simulink library "APST_Lib"  (R2016a)
settings: Solver=ode45  StartTime=0.0  StopTime=10.0  RelTol=1e-3
undefined symbols (not defined in the file or in its folder): ACM, COMP_MAP, rev_comms_sink
libraries: APST_Lib x97
(part 5 of 6)

== system APST_Lib/Electrical Components/Load ==
  In1 : Inport
  In2 : Inport  Port=2
  Bus Selector : BusSelector  OutputSignals=V,I
  Constant : Constant  Value=0
  Constant1 : Constant  Value=0
  Data_Sink1 : APST_Lib/Support Components/Data_Sink
  Divide : Product  Inputs=/
  Gain : Gain  Gain=1000
  P : Constant  Value=P_max
  Product : Product
  Product1 : Product
  Sink1 : APST_Lib/Support Components/Sink
  Switch : Switch  Criteria=u2 > Threshold
  Switch1 : Switch  Criteria=u2 > Threshold
  Terminator3 : Terminator
  b1 : BusCreator  Inputs=1
  wires:
  Bus Selector/1 -> Switch1/2, Divide/1, Switch/2  "<V>"
  Bus Selector/2 -> Terminator3/1  "<I>"
  Product1/1 -> Gain/1  "I"
  In1/1 -> Bus Selector/1
  P/1 -> Product/1
  In2/1 -> Product/2
  Switch/1 -> Product1/1
  Divide/1 -> Switch/1
  Constant/1 -> Switch/3
  b1/1 -> Data_Sink1/1
  Switch1/1 -> b1/1, Product1/2  "Power"
  Constant1/1 -> Switch1/3
  Product/1 -> Switch1/1  "Power"
  Gain/1 -> Sink1/1

== system APST_Lib/Electrical Components/QLoad ==
  In1 : Inport
  In2 : Inport  Port=2
  Bus Selector : BusSelector  OutputSignals=V,I
  Constant : Constant  Value=0
  Constant1 : Constant  Value=0
  Data_Sink1 : APST_Lib/Support Components/Data_Sink
  Divide : Product  Inputs=/
  Divide1 : Product  Inputs=*/
  Fcn : Fcn  Expr=1-u
  Gain : Gain  Gain=1000
  P : Constant  Value=P_max
  Product : Product
  Product1 : Product
  Product2 : Product
  Sink1 : APST_Lib/Support Components/Sink
  Source1 : APST_Lib/Support Components/Source
  Switch : Switch  Criteria=u2 > Threshold
  Switch1 : Switch  Criteria=u2 > Threshold
  Terminator3 : Terminator
  b1 : BusCreator  Inputs=3
  b2 : BusCreator  Inputs=2
  eta : Fcn  Expr=a*u^2+b*u+c
  Out1 : Outport
  wires:
  Bus Selector/1 -> Divide/1, Switch/2, Switch1/2  "<V>"
  Bus Selector/2 -> Terminator3/1  "<I>"
  Product1/1 -> Gain/1  "I"
  In1/1 -> Bus Selector/1
  P/1 -> Product/1
  In2/1 -> Product/2
  Switch/1 -> Product1/1
  Divide/1 -> Switch/1
  Constant/1 -> Switch/3
  b1/1 -> Data_Sink1/1
  Switch1/1 -> b1/2, Divide1/1  "Power"
  b2/1 -> Out1/1
  [T] -> b2/1  "T"
  [Q] -> b2/2  "Q_kW"
  Source1/1 -> [T]
  [T] -> eta/1
  eta/1 -> b1/1, Fcn/1, Divide1/2  "eta"
  Divide1/1 -> Product1/2, Product2/1  "P_in"
  Product2/1 -> [Q]
  Fcn/1 -> Product2/2
  Constant1/1 -> Switch1/3
  Product/1 -> Switch1/1  "Power"
  [Q] -> b1/3  "Q_kW"
  Gain/1 -> Sink1/1

== system APST_Lib/Electrical Components/Switch ==
  In : Inport
  u : Inport  Port=2
  Bus Creator1 : BusCreator  Inputs=2
  Bus Selector : BusSelector  OutputSignals=V,I
  Product : Product
  Product1 : Product
  Sink1 : APST_Lib/Support Components/Sink
  Source1 : APST_Lib/Support Components/Source
  Terminator3 : Terminator
  Out : Outport
  wires:
  Product/1 -> Bus Creator1/1  "V"
  Bus Creator1/1 -> Out/1
  In/1 -> Bus Selector/1
  Product1/1 -> Sink1/1, Bus Creator1/2  "I"
  Bus Selector/2 -> Terminator3/1  "<I>"
  Bus Selector/1 -> Product/1  "<V>"
  u/1 -> Product1/1, Product/2
  Source1/1 -> Product1/2  "I"

== system APST_Lib/Source & Sinks/Flow Flow Source (Pressure) ==
  In2 : Inport
  In3 : Inport  Port=2
  Constant4 : Constant  Value=-1
  Source1 : Subsystem  mask(Source){}
      mask help: Used for receiving data from the downstream component.
      mask init:
      | n_src = gcb;
      | n_src = str2num(n_src(end));
      | try
      |     rev_comms_source(n_src);
      | catch
      | 
      | end
      mask Display: text(0.25,0.5,'Source')
  Terminator : Terminator
  b1 : BusCreator  Inputs=3
  Out1 : Outport
  wires:
  b1/1 -> Out1/1
  Constant4/1 -> b1/1  "mdot_kgps"
  In2/1 -> b1/2  "T_C"
  In3/1 -> b1/3  "P_kPa"
  Source1/1(Out1) -> Terminator/1

== system APST_Lib/Source & Sinks/Flow Sink (Generic) ==
  In4 : Inport
  In3 : Inport  Port=2
  Sink1 : APST_Lib/Support Components/Sink
  Terminator : Terminator
  wires:
  In3/1 -> Sink1/1
  In4/1 -> Terminator/1

== system APST_Lib/Source & Sinks/Flow Sink (Mass Flow Rate) ==
  In4 : Inport
  In3 : Inport  Port=2
  Sink1 : APST_Lib/Support Components/Sink
  Terminator : Terminator
  wires:
  In3/1 -> Sink1/1  "mdot_kgps"
  In4/1 -> Terminator/1

== system APST_Lib/Source & Sinks/Flow Sink (Pressure) ==
  In4 : Inport
  In3 : Inport  Port=2
  Sink1 : APST_Lib/Support Components/Sink
  Terminator : Terminator
  wires:
  In3/1 -> Sink1/1  "P_kPa"
  In4/1 -> Terminator/1

== system APST_Lib/Source & Sinks/Flow Source (Mass Flow Rate) ==
  In1 : Inport
  In2 : Inport  Port=2
  Constant4 : Constant  Value=-1
  Source1 : Subsystem  mask(Source){}
      mask help: Used for receiving data from the downstream component.
      mask init:
      | n_src = gcb;
      | n_src = str2num(n_src(end));
      | try
      |     rev_comms_source(n_src);
      | catch
      | 
      | end
      mask Display: text(0.25,0.5,'Source')
  Terminator : Terminator
  b1 : BusCreator  Inputs=3
  Out1 : Outport
  wires:
  b1/1 -> Out1/1
  In1/1 -> b1/2  "T_C"
  In2/1 -> b1/1  "mdot_kgps"
  Constant4/1 -> b1/3  "P_kPa"
  Source1/1(Out1) -> Terminator/1

== system APST_Lib/Support Components/Data Manager ==
  Data : Outport

== system APST_Lib/Support Components/Data_Sink ==
  " " : Inport
  tag scope: gdata_SupportComponentsData_Sink=global
  wires:
  " "/1 -> [gdata_SupportComponentsData_Sink]

== system APST_Lib/Support Components/Sink ==
  In1 : Inport
  tag scope: gdata_APST_LibSupportComponentsSink=global
  wires:
  In1/1 -> [gdata_APST_LibSupportComponentsSink]

== system APST_Lib/Support Components/Source ==
  Out1 : Outport
  wires:
  [gdata_Thermal_System_BUSM2FSink2] -> Out1/1

== system APST_Lib/Support Components/Unit Conversion  ==
  Signal_in : Inport
  conv_fcn : Fcn  Expr=(u(1)+459.67)/1.8-273.15
  Converted Signal Out : Outport
  wires:
  conv_fcn/1 -> Converted Signal Out/1
  Signal_in/1 -> conv_fcn/1

== system APST_Lib/Thermal Components/ACM Shaft  ==
  Power In/Out [vector] : Inport
  Bus Creator2 : BusCreator  Inputs=1
  Comp Inertia : Constant  Value=J_comp
  Data_Sink : APST_Lib/Support Components/Data_Sink
  Divide : Product  Inputs=*//
  Integrator : Integrator  InitialCondition=N_init * 2 * pi / 60 + eps  LimitOutput=on  LowerSaturationLimit=1e-3
  Mux : Mux
  Pwr Turb Inertia : Constant  Value=J_pcomp
  Shaft Inertia : Constant  Value=J_shaft
  Sum of Elements : Sum  Inputs=+
  Sum of Elements1 : Sum  Inputs=+
  Turb Inertia : Constant  Value=J_turb
  rad 2 rev : Gain  Gain=60/(2*pi)
  rad 2 rev1 : Gain  Gain=60/2/pi
  RPM : Outport
  wires:
  rad 2 rev/1 -> RPM/1
  Integrator/1 -> rad 2 rev/1, Divide/3, rad 2 rev1/1  "omega (rad/s)"
  Power In/Out [vector]/1 -> Sum of Elements/1
  Sum of Elements/1 -> Divide/1
  Divide/1 -> Integrator/1
  Sum of Elements1/1 -> Divide/2
  Shaft Inertia/1 -> Mux/1
  Comp Inertia/1 -> Mux/2
  Turb Inertia/1 -> Mux/3
  Pwr Turb Inertia/1 -> Mux/4
  Mux/1 -> Sum of Elements1/1
  rad 2 rev1/1 -> Bus Creator2/1  "RPM"
  Bus Creator2/1 -> Data_Sink/1

== system APST_Lib/Thermal Components/Air Volume ==
  In1 : Inport
  In2 : Inport  Port=2
  In3 : Inport  Port=3
  Air_Volume : MATLAB Function  TreatAsAtomicUnit=on
  Bus Creator2 : BusCreator  Inputs=3
  Bus Selector : BusSelector  OutputSignals=Q_kW
  Constant : Constant  Value=P_init
  Constant1 : Constant  Value=T_init
  Data_Sink1 : APST_Lib/Support Components/Data_Sink
  Demux : Demux  Outputs=3
  Integrate : Integrator  InitialCondition=[T_init P_init M_init]  LimitOutput=on
  Sink1 : APST_Lib/Support Components/Sink
  Sink2 : APST_Lib/Support Components/Sink  Commented=on
  Source1 : APST_Lib/Support Components/Source
  Terminator : Terminator
  b1 : BusCreator  Inputs=3
  gb1 : BusSelector  OutputSignals=mdot_kgps,T_C,P_kPa
  kW to W : Gain  Gain=1e3
  n-D Lookup Table1 : Lookup_n-D  BreakpointsForDimension1=Fluid.P  BreakpointsForDimension2=Fluid.T  BreakpointsForDimension3=[5, 7]  Table=Fluid.C_pt  ExtrapMethod=Clip  UseLastTableValue=on  RndMeth=Simplest  InputSameDT=on
  n-D Lookup Table2 : Lookup_n-D  BreakpointsForDimension1=Fluid.P  BreakpointsForDimension2=Fluid.T  BreakpointsForDimension3=[5, 7]  Table=Fluid.Rho_pt  ExtrapMethod=Clip  UseLastTableValue=on  RndMeth=Simplest  InputSameDT=on
  pout1 : From  Commented=on  GotoTag=T_tank
  Out1 : Outport
  wires:
  b1/1 -> Out1/1
  [Mdot_out] -> b1/1  "mdot_kgps"
  gb1/2 -> [T_in]  "<T_C>"
  [T_tank] -> b1/2  "T_C"
  gb1/1 -> [Mdot_in]  "<mdot_kgps>"
  In1/1 -> gb1/1
  [P_tank] -> b1/3  "P_kPa"
  gb1/3 -> Terminator/1  "<P_kPa>"
  [P_tank] -> Sink1/1
  Source1/1 -> [Mdot_out]
  In2/1 -> [T_amb]
  [Mdot_in] -> Air_Volume/2(Mdot_in)
  [Mdot_out] -> Air_Volume/3(Mdot_out)
  Air_Volume/1(x_dot) -> Integrate/1
  Integrate/1 -> Air_Volume/1(x), Demux/1
  Demux/1 -> [T_tank]
  Demux/2 -> [P_tank]
  Constant1/1 -> n-D Lookup Table2/2, n-D Lookup Table1/2
  Constant/1 -> n-D Lookup Table2/1, n-D Lookup Table1/1
  n-D Lookup Table1/1 -> Air_Volume/6(Cp)
  n-D Lookup Table2/1 -> Air_Volume/7(Rho)
  [T_in] -> Air_Volume/4(T_in)
  [T_amb] -> Air_Volume/5(T_amb)
  Bus Creator2/1 -> Data_Sink1/1
  [T_tank] -> Bus Creator2/1  "T"
  [P_tank] -> Bus Creator2/2  "P"
  [M_tank] -> Bus Creator2/3  "M"
  In3/1 -> Bus Selector/1
  kW to W/1 -> Air_Volume/8(Q)
  Demux/3 -> [M_tank]
  Bus Selector/1 -> kW to W/1  "<Q_kW>"
  pout1/1 -> Sink2/1

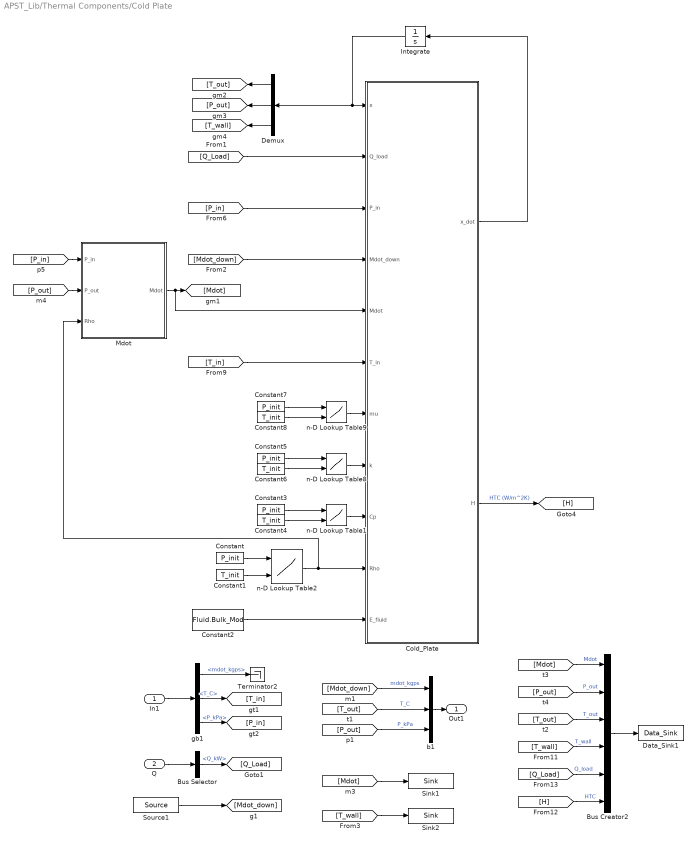
== system APST_Lib/Thermal Components/Cold Plate ==
  In1 : Inport
  Q : Inport  Port=2
  Bus Creator2 : BusCreator  Inputs=6
  Bus Selector : BusSelector  OutputSignals=Q_kW
  Cold_Plate : MATLAB Function  TreatAsAtomicUnit=on
  Constant{,3,5,7} (4 alike) : Constant  Value=P_init
  Constant{1,4,6,8} (4 alike) : Constant  Value=T_init
  Constant2 : Constant  Value=Fluid.Bulk_Mod
  Data_Sink1 : APST_Lib/Support Components/Data_Sink
  Demux : Demux  Outputs=3
  Integrate : Integrator  InitialCondition=[T_init P_init Tw_init]
  Mdot : MATLAB Function  TreatAsAtomicUnit=on
  Sink1 : APST_Lib/Support Components/Sink
  Sink2 : APST_Lib/Support Components/Sink
  Source1 : APST_Lib/Support Components/Source
  Terminator2 : Terminator
  b1 : BusCreator  Inputs=3
  gb1 : BusSelector  OutputSignals=mdot_kgps,T_C,P_kPa
  n-D Lookup Table1 : Lookup_n-D  BreakpointsForDimension1=Fluid.P  BreakpointsForDimension2=Fluid.T  BreakpointsForDimension3=[5, 7]  Table=Fluid.C_pt  ExtrapMethod=Clip  UseLastTableValue=on  RndMeth=Simplest  InputSameDT=on
  n-D Lookup Table2 : Lookup_n-D  BreakpointsForDimension1=Fluid.P  BreakpointsForDimension2=Fluid.T  BreakpointsForDimension3=[5, 7]  Table=Fluid.Rho_pt  ExtrapMethod=Clip  UseLastTableValue=on  RndMeth=Simplest  InputSameDT=on
  n-D Lookup Table8 : Lookup_n-D  BreakpointsForDimension1=Fluid.P  BreakpointsForDimension2=Fluid.T  BreakpointsForDimension3=[5, 7]  Table=Fluid.K_pt  ExtrapMethod=Clip  UseLastTableValue=on  RndMeth=Simplest  InputSameDT=on
  n-D Lookup Table9 : Lookup_n-D  BreakpointsForDimension1=Fluid.P  BreakpointsForDimension2=Fluid.T  BreakpointsForDimension3=[5, 7]  Table=Fluid.Mu_pt  ExtrapMethod=Clip  UseLastTableValue=on  RndMeth=Simplest  InputSameDT=on
  Out1 : Outport
  wires:
  Q/1 -> Bus Selector/1
  b1/1 -> Out1/1
  [Mdot_down] -> b1/1  "mdot_kgps"
  gb1/2 -> [T_in]  "<T_C>"
  [T_out] -> b1/2  "T_C"
  gb1/1 -> Terminator2/1  "<mdot_kgps>"
  In1/1 -> gb1/1
  [P_out] -> b1/3  "P_kPa"
  gb1/3 -> [P_in]  "<P_kPa>"
  [Mdot] -> Sink1/1
  [Q_Load] -> Cold_Plate/2(Q_load)
  Source1/1 -> [Mdot_down]
  [T_in] -> Cold_Plate/6(T_in)
  Cold_Plate/1(x_dot) -> Integrate/1
  Bus Creator2/1 -> Data_Sink1/1
  [T_wall] -> Bus Creator2/4  "T_wall"
  [T_out] -> Bus Creator2/3  "T_out"
  [P_out] -> Bus Creator2/2  "P_out"
  [Q_Load] -> Bus Creator2/5  "Q_load"
  [Mdot] -> Bus Creator2/1  "Mdot"
  Cold_Plate/2(H) -> [H]  "HTC (W/m^2K)"
  [H] -> Bus Creator2/6  "HTC"
  n-D Lookup Table8/1 -> Cold_Plate/8(k)
  n-D Lookup Table9/1 -> Cold_Plate/7(mu)
  Integrate/1 -> Cold_Plate/1(x), Demux/1
  n-D Lookup Table1/1 -> Cold_Plate/9(Cp)
  Constant2/1 -> Cold_Plate/11(E_fluid)
  [Mdot_down] -> Cold_Plate/4(Mdot_down)
  [P_in] -> Cold_Plate/3(P_in)
  n-D Lookup Table2/1 -> Mdot/3(Rho), Cold_Plate/10(Rho)
  Mdot/1(Mdot) -> [Mdot], Cold_Plate/5(Mdot)
  [P_in] -> Mdot/1(P_in)
  [P_out] -> Mdot/2(P_out)
  Demux/2 -> [P_out]
  Demux/1 -> [T_out]
  Demux/3 -> [T_wall]
  Constant1/1 -> n-D Lookup Table2/2
  Constant/1 -> n-D Lookup Table2/1
  Constant3/1 -> n-D Lookup Table1/1
  Constant4/1 -> n-D Lookup Table1/2
  Constant8/1 -> n-D Lookup Table9/2
  Constant5/1 -> n-D Lookup Table8/1
  Constant6/1 -> n-D Lookup Table8/2
  Constant7/1 -> n-D Lookup Table9/1
  Bus Selector/1 -> [Q_Load]  "<Q_kW>"
  [T_wall] -> Sink2/1

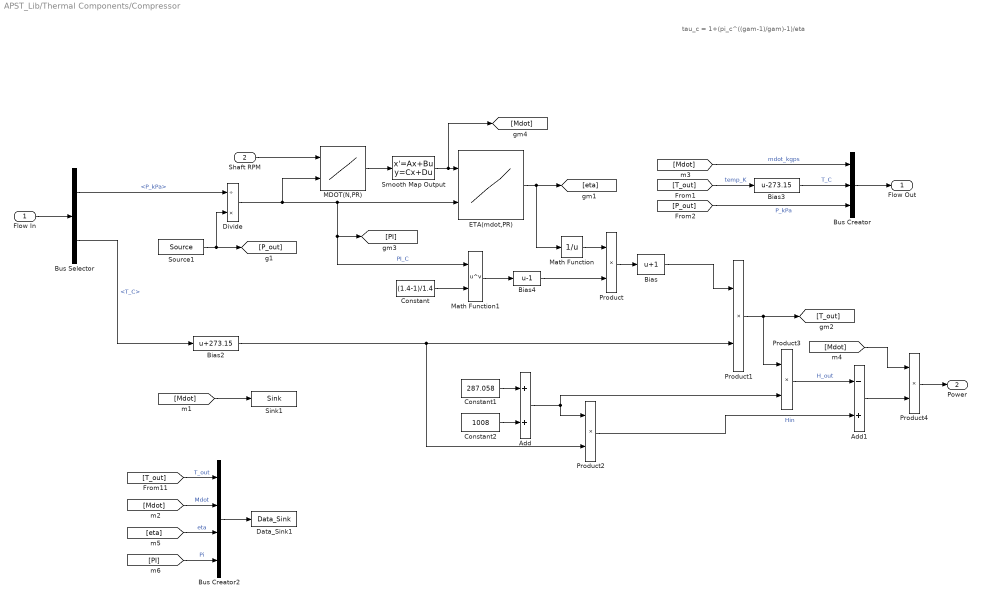
== system APST_Lib/Thermal Components/Compressor ==
  note: tau_c = 1+(pi_c^((gam-1)/gam)-1)/eta
  Flow In : Inport
  Shaft RPM : Inport  Port=2
  Add : Sum
  Add1 : Sum  Inputs=-+
  Bias : Bias  Bias=1
  Bias2 : Bias  Bias=273.15
  Bias3 : Bias  Bias=-273.15
  Bias4 : Bias  Bias=-1
  Bus Creator : BusCreator  Inputs=3
  Bus Creator2 : BusCreator  Inputs=4
  Bus Selector : BusSelector  OutputSignals=P_kPa,T_C
  Constant : Constant  Value=(1.4-1)/1.4
  Constant1 : Constant  Value=287.058
  Constant2 : Constant  Value=1008
  Data_Sink1 : APST_Lib/Support Components/Data_Sink
  Divide : Product  Inputs=/*
  ETA(mdot,PR) : Lookup_n-D  BreakpointsForDimension1=COMP.MDOT_VEC  BreakpointsForDimension2=COMP.PR_VEC  Table=COMP.ETA  ExtrapMethod=Clip  UseLastTableValue=on  InternalRulePriority=Speed  RndMeth=Simplest  InputSameDT=on
  MDOT(N,PR) : Lookup_n-D  BreakpointsForDimension1=COMP.N_VEC  BreakpointsForDimension2=COMP.PR_VEC  Table=COMP.MDOT  ExtrapMethod=Clip  UseLastTableValue=on  InternalRulePriority=Speed  RndMeth=Simplest  InputSameDT=on
  Math Function : Math  Operator=reciprocal  SaturateOnIntegerOverflow=on
  Math Function1 : Math  Operator=pow  SaturateOnIntegerOverflow=on
  Product{,1..4} (5 alike) : Product
  Sink1 : APST_Lib/Support Components/Sink
  Smooth Map Output : StateSpace  A=-50  C=50  D=0  X0=init_mdot/50
  Source1 : APST_Lib/Support Components/Source
  Flow Out : Outport
  Power : Outport  Port=2
  wires:
  MDOT(N,PR)/1 -> Smooth Map Output/1
  Shaft RPM/1 -> MDOT(N,PR)/1
  Divide/1 -> ETA(mdot,PR)/2, [PI], Math Function1/1, MDOT(N,PR)/2  "PI_C"
  Source1/1 -> Divide/2, [P_out]
  ETA(mdot,PR)/1 -> Math Function/1, [eta]
  [Mdot] -> Sink1/1
  Bus Creator2/1 -> Data_Sink1/1
  Flow In/1 -> Bus Selector/1
  Bus Selector/1 -> Divide/1  "<P_kPa>"
  Math Function/1 -> Product/1
  Product/1 -> Bias/1
  Bus Selector/2 -> Bias2/1  "<T_C>"
  Product1/1 -> [T_out], Product3/1
  Bus Creator/1 -> Flow Out/1
  [Mdot] -> Bus Creator/1  "mdot_kgps"
  [T_out] -> Bias3/1  "temp_K"
  [P_out] -> Bus Creator/3  "P_kPa"
  Constant1/1 -> Add/1
  Constant2/1 -> Add/2
  Add/1 -> Product3/2, Product2/1
  Product2/1 -> Add1/2  "Hin"
  Product3/1 -> Add1/1  "H_out"
  Add1/1 -> Product4/2
  [Mdot] -> Product4/1
  Product4/1 -> Power/1
  Bias2/1 -> Product2/2, Product1/2
  Bias3/1 -> Bus Creator/2  "T_C"
  Bias/1 -> Product1/1
  Constant/1 -> Math Function1/2
  Math Function1/1 -> Bias4/1
  Bias4/1 -> Product/2
  [Mdot] -> Bus Creator2/2  "Mdot"
  [T_out] -> Bus Creator2/1  "T_out"
  [eta] -> Bus Creator2/3  "eta"
  [PI] -> Bus Creator2/4  "Pi"
  Smooth Map Output/1 -> [Mdot], ETA(mdot,PR)/1

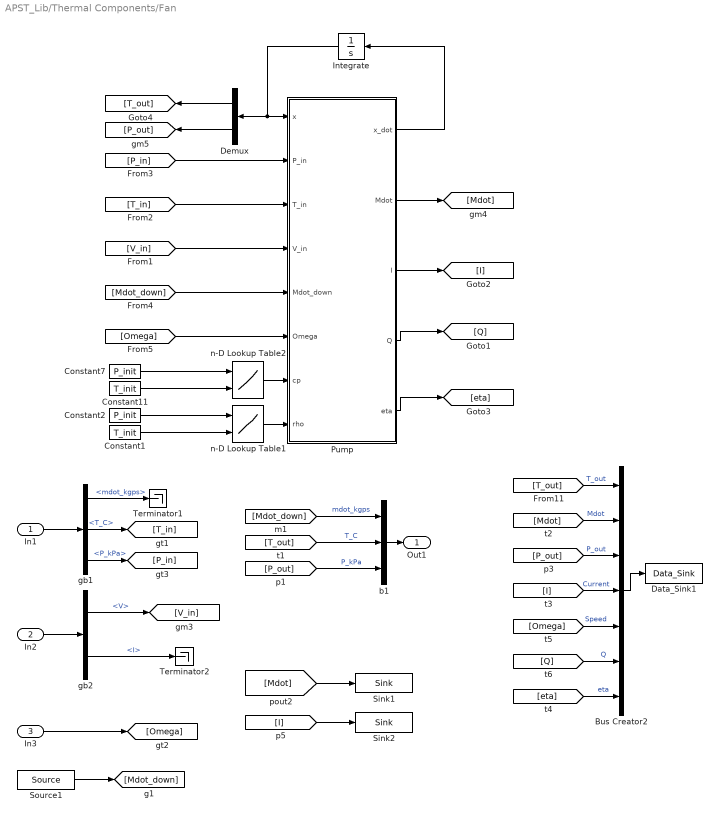
== system APST_Lib/Thermal Components/Fan ==
  In1 : Inport
  In2 : Inport  Port=2
  In3 : Inport  Port=3
  Bus Creator2 : BusCreator  Inputs=7
  Constant1 : Constant  Value=T_init
  Constant11 : Constant  Value=T_init
  Constant2 : Constant  Value=P_init
  Constant7 : Constant  Value=P_init
  Data_Sink1 : APST_Lib/Support Components/Data_Sink
  Demux : Demux  Outputs=2
  Integrate : Integrator  InitialCondition=[T_init P_init]
  Pump : MATLAB Function  TreatAsAtomicUnit=on
  Sink1 : APST_Lib/Support Components/Sink
  Sink2 : APST_Lib/Support Components/Sink
  Source1 : APST_Lib/Support Components/Source
  Terminator1 : Terminator
  Terminator2 : Terminator
  b1 : BusCreator  Inputs=3
  gb1 : BusSelector  OutputSignals=mdot_kgps,T_C,P_kPa
  gb2 : BusSelector  OutputSignals=V,I
  n-D Lookup Table1 : Lookup_n-D  BreakpointsForDimension1=Fluid.P  BreakpointsForDimension2=Fluid.T  BreakpointsForDimension3=[5, 7]  Table=Fluid.Rho_pt  ExtrapMethod=Clip  UseLastTableValue=on  RndMeth=Simplest  InputSameDT=on
  n-D Lookup Table2 : Lookup_n-D  BreakpointsForDimension1=Fluid.P  BreakpointsForDimension2=Fluid.T  BreakpointsForDimension3=[5, 7]  Table=Fluid.C_pt  ExtrapMethod=Clip  UseLastTableValue=on  RndMeth=Simplest  InputSameDT=on
  Out1 : Outport
  wires:
  b1/1 -> Out1/1
  [Mdot_down] -> b1/1  "mdot_kgps"
  gb1/2 -> [T_in]  "<T_C>"
  [T_out] -> b1/2  "T_C"
  gb1/1 -> Terminator1/1  "<mdot_kgps>"
  In1/1 -> gb1/1
  [P_out] -> b1/3  "P_kPa"
  gb1/3 -> [P_in]  "<P_kPa>"
  [Mdot] -> Sink1/1
  Source1/1 -> [Mdot_down]
  In3/1 -> [Omega]
  [Omega] -> Pump/6(Omega)
  Pump/3(I) -> [I]
  Bus Creator2/1 -> Data_Sink1/1
  [T_out] -> Bus Creator2/1  "T_out"
  [Mdot] -> Bus Creator2/2  "Mdot"
  [I] -> Bus Creator2/4  "Current"
  [P_in] -> Pump/2(P_in)
  [Mdot_down] -> Pump/5(Mdot_down)
  Integrate/1 -> Demux/1, Pump/1(x)
  Pump/1(x_dot) -> Integrate/1
  [T_in] -> Pump/3(T_in)
  [P_out] -> Bus Creator2/3  "P_out"
  Pump/2(Mdot) -> [Mdot]
  Demux/2 -> [P_out]
  Demux/1 -> [T_out]
  gb2/1 -> [V_in]  "<V>"
  In2/1 -> gb2/1
  gb2/2 -> Terminator2/1  "<I>"
  [I] -> Sink2/1
  [Omega] -> Bus Creator2/5  "Speed"
  [Q] -> Bus Creator2/6  "Q"
  Pump/4(Q) -> [Q]
  [V_in] -> Pump/4(V_in)
  Pump/5(eta) -> [eta]
  [eta] -> Bus Creator2/7  "eta"
  Constant7/1 -> n-D Lookup Table2/1
  Constant11/1 -> n-D Lookup Table2/2
  Constant2/1 -> n-D Lookup Table1/1
  Constant1/1 -> n-D Lookup Table1/2
  n-D Lookup Table1/1 -> Pump/8(rho)
  n-D Lookup Table2/1 -> Pump/7(cp)

== system APST_Lib/Thermal Components/Flow Split_Junction ==
  In1 : Inport
  Bus Creator2 : BusCreator  Inputs=2
  Constant11 : Constant  Value=T_init
  Constant5 : Constant  Value=Fluid.Bulk_Mod
  Constant7 : Constant  Value=P_init
  Data_Sink1 : APST_Lib/Support Components/Data_Sink
  Demux : Demux  Outputs=2
  Dynamic_Flow_Split_Junction : MATLAB Function  TreatAsAtomicUnit=on
  Integrator1 : Integrator  InitialCondition=[T_init P_init]
  Mux_In_1 : Mux  Inputs=1
  Mux_In_2 : Mux  Inputs=1
  Mux_In_3 : Mux  Inputs=1
  Selector1 : Selector  InputPortWidth=1  IndexOptions=Index vector (dialog)  Indices=[1 ]  OutputSizes=1
  Selector2 : Selector  InputPortWidth=1  IndexOptions=Index vector (dialog)  Indices=[1 ]  OutputSizes=1
  Sink1 : APST_Lib/Support Components/Sink
  Source1 : APST_Lib/Support Components/Source
  b1 : BusCreator  Inputs=3
  gb1 : BusSelector  OutputSignals=mdot_kgps,T_C,P_kPa
  gp1 : Terminator
  n-D Lookup Table2 : Lookup_n-D  BreakpointsForDimension1=Fluid.P  BreakpointsForDimension2=Fluid.T  BreakpointsForDimension3=[5, 7]  Table=Fluid.Rho_pt  ExtrapMethod=Clip  UseLastTableValue=on  RndMeth=Simplest  InputSameDT=on
  Out1 : Outport
  wires:
  b1/1 -> Out1/1
  [M_out1] -> b1/1  "mdot_kgps"
  gb1/2 -> [T_in1]  "<T_C>"
  [T] -> b1/2  "T_C"
  gb1/1 -> [M_in1]  "<mdot_kgps>"
  Source1/1 -> [M_out1]
  In1/1 -> gb1/1
  [P] -> b1/3  "P_kPa"
  gb1/3 -> gp1/1  "<P_kPa>"
  Mux_In_3/1 -> Selector2/1
  Mux_In_1/1 -> Selector1/1
  Mux_In_2/1 -> Dynamic_Flow_Split_Junction/3(Mdot_out)
  [M_in1] -> Mux_In_1/1
  [M_out1] -> Mux_In_2/1
  [T_in1] -> Mux_In_3/1
  [P] -> Sink1/1
  Dynamic_Flow_Split_Junction/1(x_dot) -> Integrator1/1
  Bus Creator2/1 -> Data_Sink1/1
  [T] -> Bus Creator2/1  "T_out"
  [P] -> Bus Creator2/2  "P"
  Integrator1/1 -> Demux/1, Dynamic_Flow_Split_Junction/1(x)
  Selector1/1 -> Dynamic_Flow_Split_Junction/2(Mdot_in)
  Constant5/1 -> Dynamic_Flow_Split_Junction/6(E_fluid)
  n-D Lookup Table2/1 -> Dynamic_Flow_Split_Junction/5(rho)
  Constant7/1 -> n-D Lookup Table2/1
  Constant11/1 -> n-D Lookup Table2/2
  Demux/1 -> [T]
  Demux/2 -> [P]
  Selector2/1 -> Dynamic_Flow_Split_Junction/4(T_in)

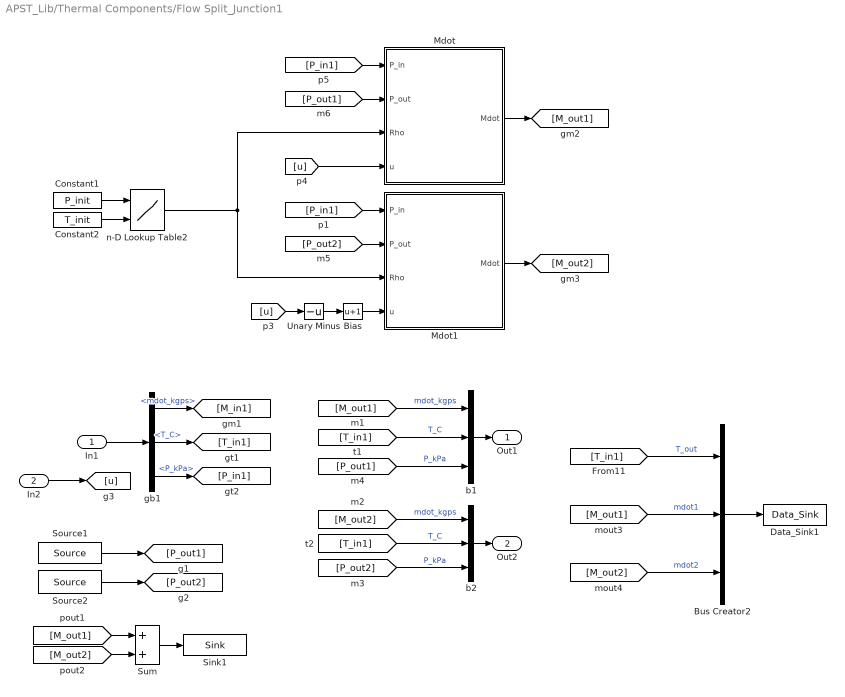
== system APST_Lib/Thermal Components/Flow Split_Junction1 ==
  In1 : Inport
  In2 : Inport  Port=2
  Bias : Bias  Bias=1
  Bus Creator2 : BusCreator  Inputs=3
  Constant1 : Constant  Value=P_init
  Constant2 : Constant  Value=T_init
  Data_Sink1 : APST_Lib/Support Components/Data_Sink
  Mdot : MATLAB Function  TreatAsAtomicUnit=on
  Mdot1 : MATLAB Function  TreatAsAtomicUnit=on
  Sink1 : APST_Lib/Support Components/Sink
  Source1 : APST_Lib/Support Components/Source
  Source2 : APST_Lib/Support Components/Source
  Sum : Sum
  Unary Minus : UnaryMinus
  b1 : BusCreator  Inputs=3
  b2 : BusCreator  Inputs=3
  gb1 : BusSelector  OutputSignals=mdot_kgps,T_C,P_kPa
  n-D Lookup Table2 : Lookup_n-D  BreakpointsForDimension1=Fluid.P  BreakpointsForDimension2=Fluid.T  BreakpointsForDimension3=[5, 7]  Table=Fluid.Rho_pt  ExtrapMethod=Clip  UseLastTableValue=on  RndMeth=Simplest  InputSameDT=on
  Out1 : Outport
  Out2 : Outport  Port=2
  wires:
  [T_in1] -> Bus Creator2/1  "T_out"
  Bus Creator2/1 -> Data_Sink1/1
  gb1/3 -> [P_in1]  "<P_kPa>"
  [P_out1] -> b1/3  "P_kPa"
  In1/1 -> gb1/1
  Source1/1 -> [P_out1]
  gb1/1 -> [M_in1]  "<mdot_kgps>"
  [T_in1] -> b1/2  "T_C"
  gb1/2 -> [T_in1]  "<T_C>"
  [M_out1] -> b1/1  "mdot_kgps"
  b1/1 -> Out1/1
  [M_out2] -> b2/1  "mdot_kgps"
  [T_in1] -> b2/2  "T_C"
  [P_out2] -> b2/3  "P_kPa"
  b2/1 -> Out2/1
  Source2/1 -> [P_out2]
  In2/1 -> [u]
  [M_out2] -> Bus Creator2/3  "mdot2"
  [M_out1] -> Bus Creator2/2  "mdot1"
  n-D Lookup Table2/1 -> Mdot/3(Rho), Mdot1/3(Rho)
  [P_in1] -> Mdot/1(P_in)
  [P_out1] -> Mdot/2(P_out)
  [P_in1] -> Mdot1/1(P_in)
  [P_out2] -> Mdot1/2(P_out)
  Mdot/1(Mdot) -> [M_out1]
  [u] -> Mdot/4(u)
  Unary Minus/1 -> Bias/1
  Bias/1 -> Mdot1/4(u)
  [u] -> Unary Minus/1
  Constant1/1 -> n-D Lookup Table2/1
  Constant2/1 -> n-D Lookup Table2/2
  Mdot1/1(Mdot) -> [M_out2]
  Sum/1 -> Sink1/1
  [M_out1] -> Sum/1
  [M_out2] -> Sum/2

== system APST_Lib/Thermal Components/Fluid Tank ==
  In1 : Inport
  In2 : Inport  Port=2
  In3 : Inport  Port=3
  Bus Creator2 : BusCreator  Inputs=3
  Constant : Constant  Value=P_init
  Constant1 : Constant  Value=T_init
  Data_Sink1 : APST_Lib/Support Components/Data_Sink
  Demux : Demux  Outputs=3
  Fuel Mass Check : Subsystem  TreatAsAtomicUnit=on
  Integrate : Integrator  InitialCondition=[T_init P_init M_init]  LimitOutput=on  LowerSaturationLimit=[-inf -inf 1e-1]  ShowSaturationPort=on
  Selector : Selector  InputPortWidth=3  IndexOptions=Index vector (dialog)  Indices=3  OutputSizes=1
  Sink1 : APST_Lib/Support Components/Sink
  Source1 : APST_Lib/Support Components/Source
  Tank : MATLAB Function  TreatAsAtomicUnit=on
  Terminator : Terminator
  b1 : BusCreator  Inputs=3
  gb1 : BusSelector  OutputSignals=mdot_kgps,T_C,P_kPa
  kW to W : Gain  Gain=1e3
  n-D Lookup Table1 : Lookup_n-D  BreakpointsForDimension1=Fluid.P  BreakpointsForDimension2=Fluid.T  BreakpointsForDimension3=[5, 7]  Table=Fluid.C_pt  ExtrapMethod=Clip  UseLastTableValue=on  RndMeth=Simplest  InputSameDT=on
  n-D Lookup Table2 : Lookup_n-D  BreakpointsForDimension1=Fluid.P  BreakpointsForDimension2=Fluid.T  BreakpointsForDimension3=[5, 7]  Table=Fluid.Rho_pt  ExtrapMethod=Clip  UseLastTableValue=on  RndMeth=Simplest  InputSameDT=on
  Out1 : Outport
  Out2 : Outport  Port=2
  wires:
  b1/1 -> Out1/1
  [Mdot_out] -> b1/1  "mdot_kgps"
  gb1/2 -> [T_in]  "<T_C>"
  [T_tank] -> b1/2  "T_C"
  gb1/1 -> [Mdot_in]  "<mdot_kgps>"
  In1/1 -> gb1/1
  [P_tank] -> b1/3  "P_kPa"
  gb1/3 -> Terminator/1  "<P_kPa>"
  [P_tank] -> Sink1/1
  Source1/1 -> [Mdot_out]
  In2/1 -> [T_amb]
  [Mdot_in] -> Tank/2(Mdot_in)
  [Mdot_out] -> Tank/3(Mdot_out)
  Tank/1(x_dot) -> Integrate/1
  Integrate/1 -> Tank/1(x), Demux/1
  Demux/1 -> [T_tank]
  Demux/2 -> [P_tank]
  Constant1/1 -> n-D Lookup Table2/2, n-D Lookup Table1/2
  Constant/1 -> n-D Lookup Table2/1, n-D Lookup Table1/1
  n-D Lookup Table1/1 -> Tank/6(Cp)
  n-D Lookup Table2/1 -> Tank/7(Rho)
  [T_in] -> Tank/4(T_in)
  [T_amb] -> Tank/5(T_amb)
  Bus Creator2/1 -> Data_Sink1/1
  [T_tank] -> Bus Creator2/1  "T_tank"
  [P_tank] -> Bus Creator2/2  "P_tank"
  [M_tank] -> Bus Creator2/3  "M_tank"
  In3/1 -> kW to W/1
  kW to W/1 -> Tank/8(Q)
  Demux/3 -> [M_tank]
  [M_tank] -> Out2/1
  Integrate/2 -> Selector/1
  Selector/1 -> Fuel Mass Check/Trigger

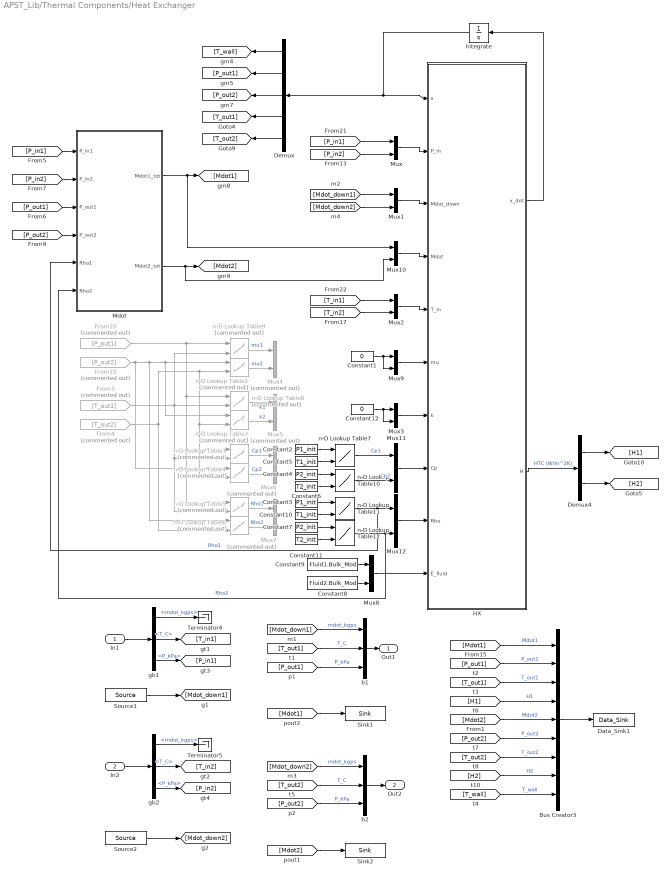
== system APST_Lib/Thermal Components/Heat Exchanger ==
  In1 : Inport
  In2 : Inport  Port=2
  Bus Creator3 : BusCreator  Inputs=9
  Constant1 : Constant  Value=0
  Constant10 : Constant  Value=T1_init
  Constant11 : Constant  Value=T2_init
  Constant12 : Constant  Value=0
  Constant2 : Constant  Value=P1_init
  Constant3 : Constant  Value=P1_init
  Constant4 : Constant  Value=P2_init
  Constant5 : Constant  Value=T1_init
  Constant6 : Constant  Value=T2_init
  Constant7 : Constant  Value=P2_init
  Constant8 : Constant  Value=Fluid2.Bulk_Mod
  Constant9 : Constant  Value=Fluid1.Bulk_Mod
  Data_Sink1 : APST_Lib/Support Components/Data_Sink
  Demux : Demux  Outputs=5
  Demux4 : Demux  Outputs=2
  From20 : From  Commented=on  GotoTag=P_out1
      settings: CloseFcn=tagdialog Close
  From25 : From  Commented=on  GotoTag=P_out2
      settings: CloseFcn=tagdialog Close
  From3 : From  Commented=on  GotoTag=T_out1
      settings: CloseFcn=tagdialog Close
  From4 : From  Commented=on  GotoTag=T_out2
      settings: CloseFcn=tagdialog Close
  HX : MATLAB Function  TreatAsAtomicUnit=on
  Integrate : Integrator  InitialCondition=[Tw_init P1_init P2_init T1_init T2_init]
  Mdot : MATLAB Function  TreatAsAtomicUnit=on
  Mux{,1..3,8..12} (9 alike) : Mux  Inputs=2
  Mux{4..7} (4 alike) : Mux  Commented=on  Inputs=2
  Sink1 : APST_Lib/Support Components/Sink
  Sink2 : APST_Lib/Support Components/Sink
  Source1 : APST_Lib/Support Components/Source
  Source2 : APST_Lib/Support Components/Source
  Terminator4 : Terminator
  Terminator5 : Terminator
  b1 : BusCreator  Inputs=3
  b2 : BusCreator  Inputs=3
  gb1 : BusSelector  OutputSignals=mdot_kgps,T_C,P_kPa
  gb2 : BusSelector  OutputSignals=mdot_kgps,T_C,P_kPa
  n-D Lookup Table1 : Lookup_n-D  Commented=on  BreakpointsForDimension1=Fluid1.P  BreakpointsForDimension2=Fluid1.T  BreakpointsForDimension3=[5, 7]  Table=Fluid1.C_pt  ExtrapMethod=Clip  RndMeth=Simplest  InputSameDT=on
  n-D Lookup Table10 : Lookup_n-D  BreakpointsForDimension1=Fluid2.P  BreakpointsForDimension2=Fluid2.T  BreakpointsForDimension3=[5, 7]  Table=Fluid2.C_pt  ExtrapMethod=Clip  UseLastTableValue=on  RndMeth=Simplest  InputSameDT=on
  n-D Lookup Table11 : Lookup_n-D  BreakpointsForDimension1=Fluid1.P  BreakpointsForDimension2=Fluid1.T  BreakpointsForDimension3=[5, 7]  Table=Fluid1.Rho_pt  ExtrapMethod=Clip  UseLastTableValue=on  RndMeth=Simplest  InputSameDT=on
  n-D Lookup Table12 : Lookup_n-D  BreakpointsForDimension1=Fluid2.P  BreakpointsForDimension2=Fluid2.T  BreakpointsForDimension3=[5, 7]  Table=Fluid2.Rho_pt  ExtrapMethod=Clip  UseLastTableValue=on  RndMeth=Simplest  InputSameDT=on
  n-D Lookup Table2 : Lookup_n-D  Commented=on  BreakpointsForDimension1=Fluid2.P  BreakpointsForDimension2=Fluid2.T  BreakpointsForDimension3=[5, 7]  Table=Fluid2.Mu_pt  ExtrapMethod=Clip  UseLastTableValue=on  RndMeth=Simplest  InputSameDT=on
  n-D Lookup Table3 : Lookup_n-D  Commented=on  BreakpointsForDimension1=Fluid2.P  BreakpointsForDimension2=Fluid2.T  BreakpointsForDimension3=[5, 7]  Table=Fluid2.K_pt  ExtrapMethod=Clip  UseLastTableValue=on  RndMeth=Simplest  InputSameDT=on
  n-D Lookup Table4 : Lookup_n-D  Commented=on  BreakpointsForDimension1=Fluid2.P  BreakpointsForDimension2=Fluid2.T  BreakpointsForDimension3=[5, 7]  Table=Fluid2.C_pt  ExtrapMethod=Clip  UseLastTableValue=on  RndMeth=Simplest  InputSameDT=on
  n-D Lookup Table5 : Lookup_n-D  Commented=on  BreakpointsForDimension1=Fluid1.P  BreakpointsForDimension2=Fluid1.T  BreakpointsForDimension3=[5, 7]  Table=Fluid1.Rho_pt  ExtrapMethod=Clip  UseLastTableValue=on  RndMeth=Simplest  InputSameDT=on
  n-D Lookup Table6 : Lookup_n-D  Commented=on  BreakpointsForDimension1=Fluid2.P  BreakpointsForDimension2=Fluid2.T  BreakpointsForDimension3=[5, 7]  Table=Fluid2.Rho_pt  ExtrapMethod=Clip  UseLastTableValue=on  RndMeth=Simplest  InputSameDT=on
  n-D Lookup Table7 : Lookup_n-D  BreakpointsForDimension1=Fluid1.P  BreakpointsForDimension2=Fluid1.T  BreakpointsForDimension3=[5, 7]  Table=Fluid1.C_pt  ExtrapMethod=Clip  RndMeth=Simplest  InputSameDT=on
  n-D Lookup Table8 : Lookup_n-D  Commented=on  BreakpointsForDimension1=Fluid1.P  BreakpointsForDimension2=Fluid1.T  BreakpointsForDimension3=[5, 7]  Table=Fluid1.K_pt  ExtrapMethod=Clip  UseLastTableValue=on  RndMeth=Simplest  InputSameDT=on
  n-D Lookup Table9 : Lookup_n-D  Commented=on  BreakpointsForDimension1=Fluid1.P  BreakpointsForDimension2=Fluid1.T  BreakpointsForDimension3=[5, 7]  Table=Fluid1.Mu_pt  ExtrapMethod=Clip  UseLastTableValue=on  RndMeth=Simplest  InputSameDT=on
  Out1 : Outport
  Out2 : Outport  Port=2
  wires:
  b1/1 -> Out1/1
  [Mdot_down1] -> b1/1  "mdot_kgps"
  gb1/2 -> [T_in1]  "<T_C>"
  [T_out1] -> b1/2  "T_C"
  gb1/1 -> Terminator4/1  "<mdot_kgps>"
  In1/1 -> gb1/1
  [P_out1] -> b1/3  "P_kPa"
  gb1/3 -> [P_in1]  "<P_kPa>"
  [Mdot1] -> Sink1/1
  [P_in1] -> Mux/1
  Source1/1 -> [Mdot_down1]
  [Mdot_down1] -> Mux1/1
  [T_in1] -> Mux2/1
  HX/1(x_dot) -> Integrate/1
  Integrate/1 -> Demux/1, HX/1(x)
  Demux/1 -> [T_wall]
  Demux/2 -> [P_out1]
  HX/2(H) -> Demux4/1  "HTC (W/m^2K)"
  n-D Lookup Table8/1 -> Mux5/1  "k1"
  n-D Lookup Table9/1 -> Mux4/1  "mu1"
  From3/1 -> n-D Lookup Table9/2, n-D Lookup Table5/2, n-D Lookup Table1/2, n-D Lookup Table8/2
  From20/1 -> n-D Lookup Table5/1, n-D Lookup Table1/1, n-D Lookup Table8/1, n-D Lookup Table9/1
  n-D Lookup Table1/1 -> Mux6/1  "Cp1"
  n-D Lookup Table11/1 -> Mux12/1, Mdot/5(Rho1)  "Rho1"
  gb2/2 -> [T_in2]  "<T_C>"
  gb2/1 -> Terminator5/1  "<mdot_kgps>"
  In2/1 -> gb2/1
  gb2/3 -> [P_in2]  "<P_kPa>"
  Source2/1 -> [Mdot_down2]
  b2/1 -> Out2/1
  [Mdot_down2] -> b2/1  "mdot_kgps"
  [T_out2] -> b2/2  "T_C"
  [P_out2] -> b2/3  "P_kPa"
  [Mdot2] -> Sink2/1
  Mux/1 -> HX/2(P_in)
  [P_in2] -> Mux/2
  Mux1/1 -> HX/3(Mdot_down)
  [Mdot_down2] -> Mux1/2
  Mux2/1 -> HX/5(T_in)
  [T_in2] -> Mux2/2
  n-D Lookup Table2/1 -> Mux4/2  "mu2"
  From25/1 -> n-D Lookup Table6/1, n-D Lookup Table3/1, n-D Lookup Table2/1, n-D Lookup Table4/1
  From4/1 -> n-D Lookup Table3/2, n-D Lookup Table4/2, n-D Lookup Table2/2, n-D Lookup Table6/2
  n-D Lookup Table3/1 -> Mux5/2  "k2"
  n-D Lookup Table4/1 -> Mux6/2  "Cp2"
  Mux8/1 -> HX/10(E_fluid)
  Demux4/1 -> [H1]
  Demux4/2 -> [H2]
  Demux/3 -> [P_out2]
  Constant9/1 -> Mux8/1
  Constant8/1 -> Mux8/2
  [H2] -> Bus Creator3/8  "H2"
  [T_out2] -> Bus Creator3/7  "T_out2"
  [P_out2] -> Bus Creator3/6  "P_out2"
  [Mdot2] -> Bus Creator3/5  "Mdot2"
  [H1] -> Bus Creator3/4  "H1"
  [T_out1] -> Bus Creator3/3  "T_out1"
  [T_wall] -> Bus Creator3/9  "T_wall"
  [P_out1] -> Bus Creator3/2  "P_out1"
  [Mdot1] -> Bus Creator3/1  "Mdot1"
  Bus Creator3/1 -> Data_Sink1/1
  [P_in1] -> Mdot/1(P_in1)
  n-D Lookup Table12/1 -> Mdot/6(Rho2), Mux12/2  "Rho2"
  [P_in2] -> Mdot/2(P_in2)
  [P_out2] -> Mdot/4(P_out2)
  Demux/4 -> [T_out1]
  Demux/5 -> [T_out2]
  Mdot/1(Mdot1_tot) -> Mux10/1, [Mdot1]
  Mux10/1 -> HX/4(Mdot)
  Mdot/2(Mdot2_tot) -> Mux10/2, [Mdot2]
  [P_out1] -> Mdot/3(P_out1)
  n-D Lookup Table7/1 -> Mux11/1  "Cp1"
  n-D Lookup Table10/1 -> Mux11/2  "Cp2"
  Constant2/1 -> n-D Lookup Table7/1
  Constant5/1 -> n-D Lookup Table7/2
  Constant4/1 -> n-D Lookup Table10/1
  Constant6/1 -> n-D Lookup Table10/2
  Constant3/1 -> n-D Lookup Table11/1
  Constant10/1 -> n-D Lookup Table11/2
  Constant7/1 -> n-D Lookup Table12/1
  Constant11/1 -> n-D Lookup Table12/2
  Constant1/1 -> Mux9/1, Mux9/2
  Mux11/1 -> HX/8(Cp)
  Mux12/1 -> HX/9(Rho)
  Mux9/1 -> HX/6(mu)
  Constant12/1 -> Mux3/2, Mux3/1
  Mux3/1 -> HX/7(k)
  n-D Lookup Table5/1 -> Mux7/1  "Rho1"
  n-D Lookup Table6/1 -> Mux7/2  "Rho2"

== system APST_Lib/Thermal Components/Pipe_P_to_M ==
  In1 : Inport
  Bus Creator2 : BusCreator  Inputs=3
  Constant2 : Constant  Value=Fluid.Bulk_Mod
  Constant7 : Constant  Value=P_init
  Constant8 : Constant  Value=T_init
  Data_Sink1 : APST_Lib/Support Components/Data_Sink
  Demux : Demux  Outputs=2
  Integrate : Integrator  InitialCondition=[T_init P_init]
  Mdot : MATLAB Function  TreatAsAtomicUnit=on
  Pipe_P_to_M : MATLAB Function  TreatAsAtomicUnit=on
  Sink1 : APST_Lib/Support Components/Sink
  Source1 : APST_Lib/Support Components/Source
  Terminator3 : Terminator
  b2 : BusCreator  Inputs=3
  gb2 : BusSelector  OutputSignals=mdot_kgps,T_C,P_kPa
  n-D Lookup Table2 : Lookup_n-D  BreakpointsForDimension1=Fluid.P  BreakpointsForDimension2=Fluid.T  BreakpointsForDimension3=[5, 7]  Table=Fluid.Rho_pt  ExtrapMethod=Clip  UseLastTableValue=on  RndMeth=Simplest  InputSameDT=on
  Out1 : Outport
  wires:
  Bus Creator2/1 -> Data_Sink1/1
  [T_out] -> Bus Creator2/1  "T_out"
  Constant8/1 -> n-D Lookup Table2/2
  Constant7/1 -> n-D Lookup Table2/1
  n-D Lookup Table2/1 -> Pipe_P_to_M/5(Rho), Mdot/3(Rho)
  [Mdot] -> Bus Creator2/2  "Mdot"
  [P_out] -> Bus Creator2/3  "P_out"
  Pipe_P_to_M/1(x_dot) -> Integrate/1
  Integrate/1 -> Pipe_P_to_M/1(x), Demux/1
  b2/1 -> Out1/1
  [Mdot_down] -> b2/1  "mdot_kgps"
  gb2/2 -> [T_in]  "<T_C>"
  [T_out] -> b2/2  "T_C"
  gb2/1 -> Terminator3/1  "<mdot_kgps>"
  In1/1 -> gb2/1
  [P_out] -> b2/3  "P_kPa"
  gb2/3 -> [P_in]  "<P_kPa>"
  [Mdot] -> Sink1/1
  Source1/1 -> [Mdot_down]
  [Mdot_down] -> Pipe_P_to_M/3(Mdot_down)
  Constant2/1 -> Pipe_P_to_M/6(E_fluid)
  [T_in] -> Pipe_P_to_M/2(T_in)
  [P_in] -> Mdot/1(P_in)
  [P_out] -> Mdot/2(P_out)
  Mdot/1(Mdot) -> Pipe_P_to_M/4(Mdot), [Mdot]
  Demux/2 -> [P_out]
  Demux/1 -> [T_out]

== system APST_Lib/Thermal Components/Pipe_P_to_P ==
  In1 : Inport
  Bus Creator2 : BusCreator  Inputs=2
  Constant8 : Constant  Value=T_init
  Data_Sink1 : APST_Lib/Support Components/Data_Sink
  Integrate1 : Integrator  InitialCondition=T_init
  Mdot : MATLAB Function  TreatAsAtomicUnit=on
  Pipe_P_to_M : MATLAB Function  TreatAsAtomicUnit=on
  Sink1 : APST_Lib/Support Components/Sink
  Source1 : APST_Lib/Support Components/Source
  Terminator2 : Terminator
  b1 : BusCreator  Inputs=3
  gb1 : BusSelector  OutputSignals=mdot_kgps,T_C,P_kPa
  n-D Lookup Table1 : Lookup_n-D  BreakpointsForDimension1=Fluid.P  BreakpointsForDimension2=Fluid.T  BreakpointsForDimension3=[5, 7]  Table=Fluid.Rho_pt  ExtrapMethod=Clip  UseLastTableValue=on  RndMeth=Simplest  InputSameDT=on
  Out1 : Outport
  wires:
  b1/1 -> Out1/1
  [Mdot] -> b1/1  "mdot_kgps"
  gb1/2 -> [T_in]  "<T_C>"
  [T_out] -> b1/2  "T_C"
  gb1/1 -> Terminator2/1  "<mdot_kgps>"
  In1/1 -> gb1/1
  [P_out] -> b1/3  "P_kPa"
  gb1/3 -> [P_in]  "<P_kPa>"
  [Mdot] -> Sink1/1
  Source1/1 -> [P_out]
  Bus Creator2/1 -> Data_Sink1/1
  [T_out] -> Bus Creator2/1  "T_out"
  [Mdot] -> Bus Creator2/2  "Mdot"
  Pipe_P_to_M/1(x_dot) -> Integrate1/1
  Integrate1/1 -> Pipe_P_to_M/1(x), [T_out]
  [T_in] -> Pipe_P_to_M/2(T_in)
  Constant8/1 -> n-D Lookup Table1/2
  [P_in] -> n-D Lookup Table1/1
  n-D Lookup Table1/1 -> Mdot/3(Rho), Pipe_P_to_M/4(Rho)
  [P_in] -> Mdot/1(P_in)
  [P_out] -> Mdot/2(P_out)
  Mdot/1(Mdot) -> [Mdot], Pipe_P_to_M/3(Mdot)

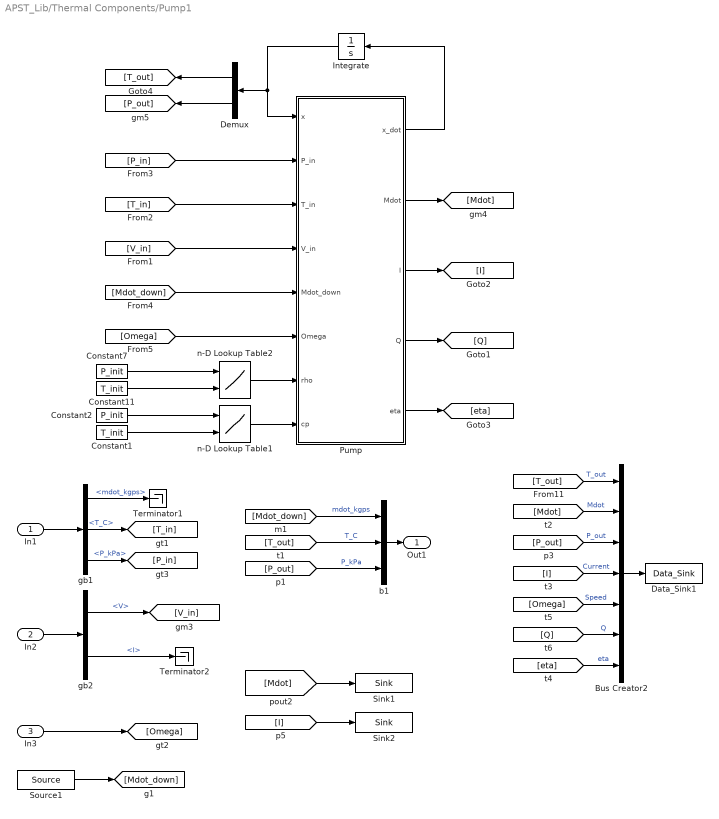
== system APST_Lib/Thermal Components/Pump1 ==
  In1 : Inport
  In2 : Inport  Port=2
  In3 : Inport  Port=3
  Bus Creator2 : BusCreator  Inputs=7
  Constant1 : Constant  Value=T_init
  Constant11 : Constant  Value=T_init
  Constant2 : Constant  Value=P_init
  Constant7 : Constant  Value=P_init
  Data_Sink1 : APST_Lib/Support Components/Data_Sink
  Demux : Demux  Outputs=2
  Integrate : Integrator  InitialCondition=[T_init P_init]
  Pump : MATLAB Function  TreatAsAtomicUnit=on
  Sink1 : APST_Lib/Support Components/Sink
  Sink2 : APST_Lib/Support Components/Sink
  Source1 : APST_Lib/Support Components/Source
  Terminator1 : Terminator
  Terminator2 : Terminator
  b1 : BusCreator  Inputs=3
  gb1 : BusSelector  OutputSignals=mdot_kgps,T_C,P_kPa
  gb2 : BusSelector  OutputSignals=V,I
  n-D Lookup Table1 : Lookup_n-D  BreakpointsForDimension1=Fluid.P  BreakpointsForDimension2=Fluid.T  BreakpointsForDimension3=[5, 7]  Table=Fluid.C_pt  ExtrapMethod=Clip  UseLastTableValue=on  RndMeth=Simplest  InputSameDT=on
  n-D Lookup Table2 : Lookup_n-D  BreakpointsForDimension1=Fluid.P  BreakpointsForDimension2=Fluid.T  BreakpointsForDimension3=[5, 7]  Table=Fluid.Rho_pt  ExtrapMethod=Clip  UseLastTableValue=on  RndMeth=Simplest  InputSameDT=on
  Out1 : Outport
  wires:
  b1/1 -> Out1/1
  [Mdot_down] -> b1/1  "mdot_kgps"
  gb1/2 -> [T_in]  "<T_C>"
  [T_out] -> b1/2  "T_C"
  gb1/1 -> Terminator1/1  "<mdot_kgps>"
  In1/1 -> gb1/1
  [P_out] -> b1/3  "P_kPa"
  gb1/3 -> [P_in]  "<P_kPa>"
  [Mdot] -> Sink1/1
  Source1/1 -> [Mdot_down]
  In3/1 -> [Omega]
  [Omega] -> Pump/6(Omega)
  Pump/3(I) -> [I]
  Bus Creator2/1 -> Data_Sink1/1
  [T_out] -> Bus Creator2/1  "T_out"
  [Mdot] -> Bus Creator2/2  "Mdot"
  [I] -> Bus Creator2/4  "Current"
  [P_in] -> Pump/2(P_in)
  [Mdot_down] -> Pump/5(Mdot_down)
  Integrate/1 -> Pump/1(x), Demux/1
  Pump/1(x_dot) -> Integrate/1
  [T_in] -> Pump/3(T_in)
  [P_out] -> Bus Creator2/3  "P_out"
  Pump/2(Mdot) -> [Mdot]
  Demux/2 -> [P_out]
  Demux/1 -> [T_out]
  gb2/1 -> [V_in]  "<V>"
  In2/1 -> gb2/1
  gb2/2 -> Terminator2/1  "<I>"
  [I] -> Sink2/1
  [Omega] -> Bus Creator2/5  "Speed"
  [Q] -> Bus Creator2/6  "Q"
  Pump/4(Q) -> [Q]
  [V_in] -> Pump/4(V_in)
  Pump/5(eta) -> [eta]
  [eta] -> Bus Creator2/7  "eta"
  Constant7/1 -> n-D Lookup Table2/1
  Constant11/1 -> n-D Lookup Table2/2
  n-D Lookup Table2/1 -> Pump/7(rho)
  Constant2/1 -> n-D Lookup Table1/1
  Constant1/1 -> n-D Lookup Table1/2
  n-D Lookup Table1/1 -> Pump/8(cp)

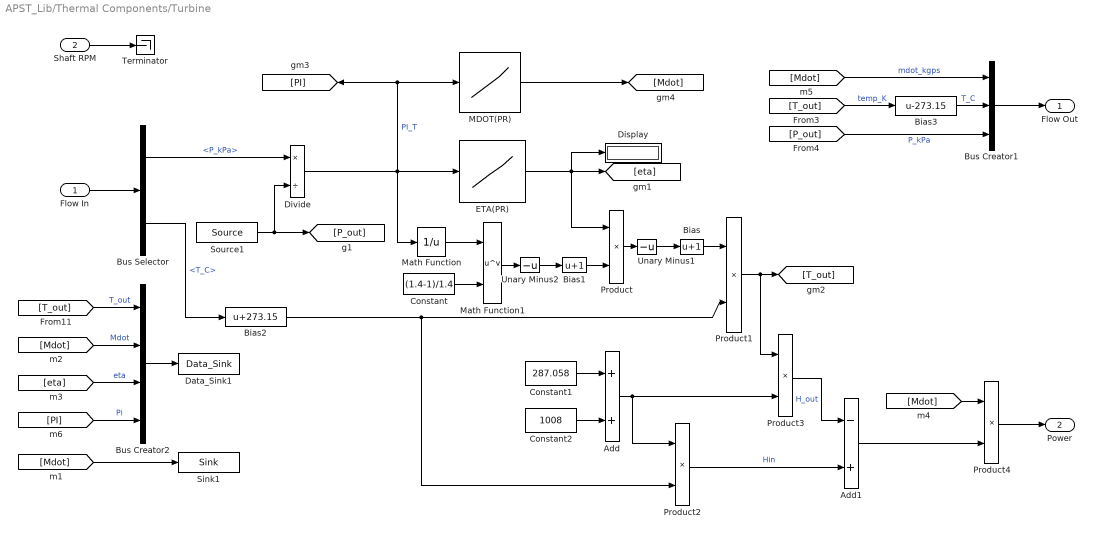
== system APST_Lib/Thermal Components/Turbine ==
  Flow In : Inport
  Shaft RPM : Inport  Port=2
  Add : Sum
  Add1 : Sum  Inputs=-+
  Bias : Bias  Bias=1
  Bias1 : Bias  Bias=1
  Bias2 : Bias  Bias=273.15
  Bias3 : Bias  Bias=-273.15
  Bus Creator1 : BusCreator  Inputs=3
  Bus Creator2 : BusCreator  Inputs=4
  Bus Selector : BusSelector  OutputSignals=P_kPa,T_C
  Constant : Constant  Value=(1.4-1)/1.4
  Constant1 : Constant  Value=287.058
  Constant2 : Constant  Value=1008
  Data_Sink1 : APST_Lib/Support Components/Data_Sink
  Display : Display
  Divide : Product  Inputs=*/
  ETA(PR) : Lookup_n-D  NumberOfTableDimensions=1  BreakpointsForDimension1=ACM.MAP.Turb.PR_VEC  BreakpointsForDimension2=COMP_MAP.PR_VEC  Table=ACM.MAP.Turb.ETA  ExtrapMethod=Clip  UseLastTableValue=on  InternalRulePriority=Speed  RndMeth=Simplest  InputSameDT=on
  MDOT(PR) : Lookup_n-D  NumberOfTableDimensions=1  BreakpointsForDimension1=TURB.PR_VEC  BreakpointsForDimension2=COMP_MAP.PR_VEC  Table=TURB.MDOT  ExtrapMethod=Clip  UseLastTableValue=on  InternalRulePriority=Speed  RndMeth=Simplest  InputSameDT=on
  Math Function : Math  Operator=reciprocal  SaturateOnIntegerOverflow=on
  Math Function1 : Math  Operator=pow  SaturateOnIntegerOverflow=on
  Product{,1..4} (5 alike) : Product
  Sink1 : APST_Lib/Support Components/Sink
  Source1 : APST_Lib/Support Components/Source
  Terminator : Terminator
  Unary Minus1 : UnaryMinus
  Unary Minus2 : UnaryMinus
  Flow Out : Outport
  Power : Outport  Port=2
  wires:
  Divide/1 -> [PI], MDOT(PR)/1, ETA(PR)/1, Math Function/1  "PI_T"
  Source1/1 -> Divide/2, [P_out]
  [Mdot] -> Sink1/1
  Bus Creator2/1 -> Data_Sink1/1
  Flow In/1 -> Bus Selector/1
  Bus Selector/1 -> Divide/1  "<P_kPa>"
  ETA(PR)/1 -> Display/1, Product/1, [eta]
  Product/1 -> Unary Minus1/1
  Bias/1 -> Product1/1
  Bus Selector/2 -> Bias2/1  "<T_C>"
  Product1/1 -> [T_out], Product3/1
  Constant/1 -> Math Function1/2
  Constant1/1 -> Add/1
  Constant2/1 -> Add/2
  Add/1 -> Product2/1, Product3/2
  Product2/1 -> Add1/2  "Hin"
  Product3/1 -> Add1/1  "H_out"
  Add1/1 -> Product4/2
  [Mdot] -> Product4/1
  Product4/1 -> Power/1
  Shaft RPM/1 -> Terminator/1
  Bus Creator1/1 -> Flow Out/1
  [Mdot] -> Bus Creator1/1  "mdot_kgps"
  [T_out] -> Bias3/1  "temp_K"
  [P_out] -> Bus Creator1/3  "P_kPa"
  Bias3/1 -> Bus Creator1/2  "T_C"
  Bias2/1 -> Product2/2, Product1/2
  Math Function1/1 -> Unary Minus2/1
  Bias1/1 -> Product/2
  Unary Minus1/1 -> Bias/1
  Unary Minus2/1 -> Bias1/1
  Math Function/1 -> Math Function1/1
  [Mdot] -> Bus Creator2/2  "Mdot"
  [T_out] -> Bus Creator2/1  "T_out"
  [eta] -> Bus Creator2/3  "eta"
  [PI] -> Bus Creator2/4  "Pi"
  MDOT(PR)/1 -> [Mdot]

== system APST_Lib/Thermal Components/Valve ==
  In1 : Inport
  In2 : Inport  Port=2
  Bus Creator2 : BusCreator  Inputs=2
  Constant : Constant  Value=0
  Data_Sink1 : APST_Lib/Support Components/Data_Sink
  Integrate1 : Integrator  InitialCondition=T_init
  Mdot : MATLAB Function  TreatAsAtomicUnit=on
  Pipe_P_to_M : MATLAB Function  TreatAsAtomicUnit=on
  Sink1 : APST_Lib/Support Components/Sink
  Source1 : APST_Lib/Support Components/Source
  Switch : Switch  Criteria=u2 > Threshold  Threshold=0.5
  Terminator2 : Terminator
  b1 : BusCreator  Inputs=3
  gb1 : BusSelector  OutputSignals=mdot_kgps,T_C,P_kPa
  n-D Lookup Table1 : Lookup_n-D  BreakpointsForDimension1=Fluid.P  BreakpointsForDimension2=Fluid.T  BreakpointsForDimension3=[5, 7]  Table=Fluid.Rho_pt  ExtrapMethod=Clip  UseLastTableValue=on  RndMeth=Simplest  InputSameDT=on
  Out1 : Outport
  wires:
  b1/1 -> Out1/1
  [Mdot] -> b1/1  "mdot_kgps"
  gb1/2 -> [T_in]  "<T_C>"
  [T_out] -> b1/2  "T_C"
  gb1/1 -> Terminator2/1  "<mdot_kgps>"
  In1/1 -> gb1/1
  [P_out] -> b1/3  "P_kPa"
  gb1/3 -> [P_in]  "<P_kPa>"
  [Mdot] -> Sink1/1
  Source1/1 -> [P_out]
  In2/1 -> [On_off]
  Bus Creator2/1 -> Data_Sink1/1
  [T_out] -> Bus Creator2/1  "T_out"
  [Mdot] -> Bus Creator2/2  "Mdot"
  Pipe_P_to_M/1(x_dot) -> Integrate1/1
  Integrate1/1 -> Pipe_P_to_M/1(x), [T_out]
  [T_in] -> Pipe_P_to_M/2(T_in)
  [T_out] -> n-D Lookup Table1/2
  [P_out] -> n-D Lookup Table1/1
  n-D Lookup Table1/1 -> Mdot/3(Rho), Pipe_P_to_M/4(Rho)
  [P_in] -> Mdot/1(P_in)
  [P_out] -> Mdot/2(P_out)
  Switch/1 -> [Mdot], Pipe_P_to_M/3(Mdot)
  Mdot/1(Mdot) -> Switch/1
  Constant/1 -> Switch/3
  [On_off] -> Switch/2

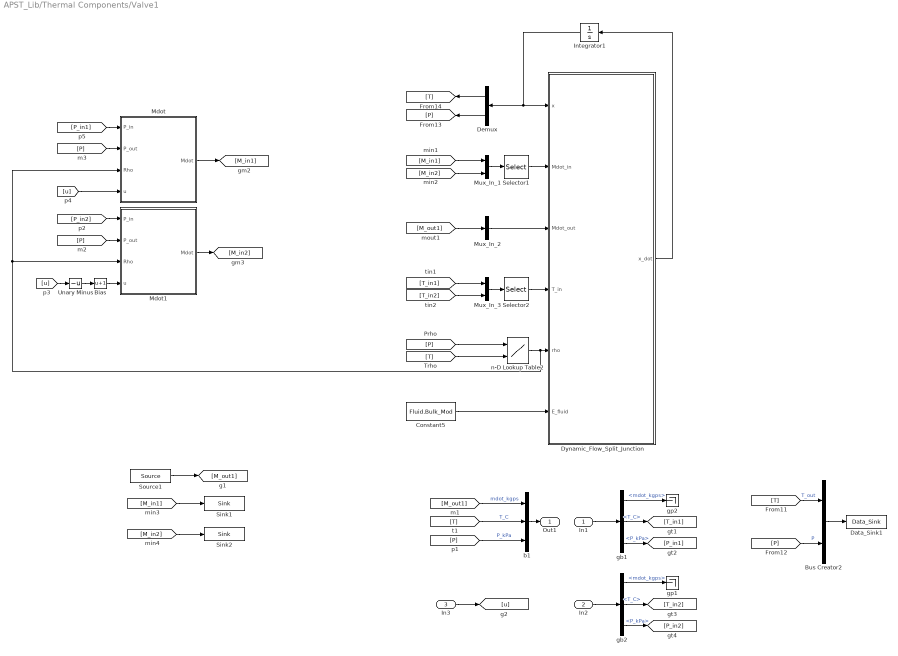
== system APST_Lib/Thermal Components/Valve1 ==
  In1 : Inport
  In2 : Inport  Port=2
  In3 : Inport  Port=3
  Bias : Bias  Bias=1
  Bus Creator2 : BusCreator  Inputs=2
  Constant5 : Constant  Value=Fluid.Bulk_Mod
  Data_Sink1 : APST_Lib/Support Components/Data_Sink
  Demux : Demux  Outputs=2
  Dynamic_Flow_Split_Junction : MATLAB Function  TreatAsAtomicUnit=on
  Integrator1 : Integrator  InitialCondition=[T_init P_init]
  Mdot : MATLAB Function  TreatAsAtomicUnit=on
  Mdot1 : MATLAB Function  TreatAsAtomicUnit=on
  Mux_In_1 : Mux  Inputs=2
  Mux_In_2 : Mux  Inputs=1
  Mux_In_3 : Mux  Inputs=2
  Selector1 : Selector  InputPortWidth=2  IndexOptions=Index vector (dialog)  Indices=[1 2 ]  OutputSizes=1
  Selector2 : Selector  InputPortWidth=2  IndexOptions=Index vector (dialog)  Indices=[1 2 ]  OutputSizes=1
  Sink1 : APST_Lib/Support Components/Sink
  Sink2 : APST_Lib/Support Components/Sink
  Source1 : APST_Lib/Support Components/Source
  Unary Minus : UnaryMinus
  b1 : BusCreator  Inputs=3
  gb1 : BusSelector  OutputSignals=mdot_kgps,T_C,P_kPa
  gb2 : BusSelector  OutputSignals=mdot_kgps,T_C,P_kPa
  gp1 : Terminator
  gp2 : Terminator
  n-D Lookup Table2 : Lookup_n-D  BreakpointsForDimension1=Fluid.P  BreakpointsForDimension2=Fluid.T  BreakpointsForDimension3=[5, 7]  Table=Fluid.Rho_pt  ExtrapMethod=Clip  UseLastTableValue=on  RndMeth=Simplest  InputSameDT=on
  Out1 : Outport
  wires:
  b1/1 -> Out1/1
  [M_out1] -> b1/1  "mdot_kgps"
  gb1/2 -> [T_in1]  "<T_C>"
  [T] -> b1/2  "T_C"
  gb1/1 -> gp2/1  "<mdot_kgps>"
  Source1/1 -> [M_out1]
  In1/1 -> gb1/1
  [P] -> b1/3  "P_kPa"
  gb1/3 -> [P_in1]  "<P_kPa>"
  Mux_In_3/1 -> Selector2/1
  Mux_In_1/1 -> Selector1/1
  Mux_In_2/1 -> Dynamic_Flow_Split_Junction/3(Mdot_out)
  [M_in1] -> Mux_In_1/1
  [M_out1] -> Mux_In_2/1
  [T_in1] -> Mux_In_3/1
  [M_in1] -> Sink1/1
  Dynamic_Flow_Split_Junction/1(x_dot) -> Integrator1/1
  Bus Creator2/1 -> Data_Sink1/1
  [T] -> Bus Creator2/1  "T_out"
  [P] -> Bus Creator2/2  "P"
  Integrator1/1 -> Demux/1, Dynamic_Flow_Split_Junction/1(x)
  Selector1/1 -> Dynamic_Flow_Split_Junction/2(Mdot_in)
  Constant5/1 -> Dynamic_Flow_Split_Junction/6(E_fluid)
  [P] -> n-D Lookup Table2/1
  [T] -> n-D Lookup Table2/2
  Demux/1 -> [T]
  Demux/2 -> [P]
  Selector2/1 -> Dynamic_Flow_Split_Junction/4(T_in)
  n-D Lookup Table2/1 -> Mdot1/3(Rho), Mdot/3(Rho), Dynamic_Flow_Split_Junction/5(rho)
  [P_in1] -> Mdot/1(P_in)
  [P] -> Mdot/2(P_out)
  [P_in2] -> Mdot1/1(P_in)
  [P] -> Mdot1/2(P_out)
  Mdot/1(Mdot) -> [M_in1]
  Mdot1/1(Mdot) -> [M_in2]
  gb2/2 -> [T_in2]  "<T_C>"
  gb2/1 -> gp1/1  "<mdot_kgps>"
  In2/1 -> gb2/1
  gb2/3 -> [P_in2]  "<P_kPa>"
  [T_in2] -> Mux_In_3/2
  [M_in2] -> Mux_In_1/2
  In3/1 -> [u]
  [u] -> Mdot/4(u)
  Unary Minus/1 -> Bias/1
  Bias/1 -> Mdot1/4(u)
  [u] -> Unary Minus/1
  [M_in2] -> Sink2/1

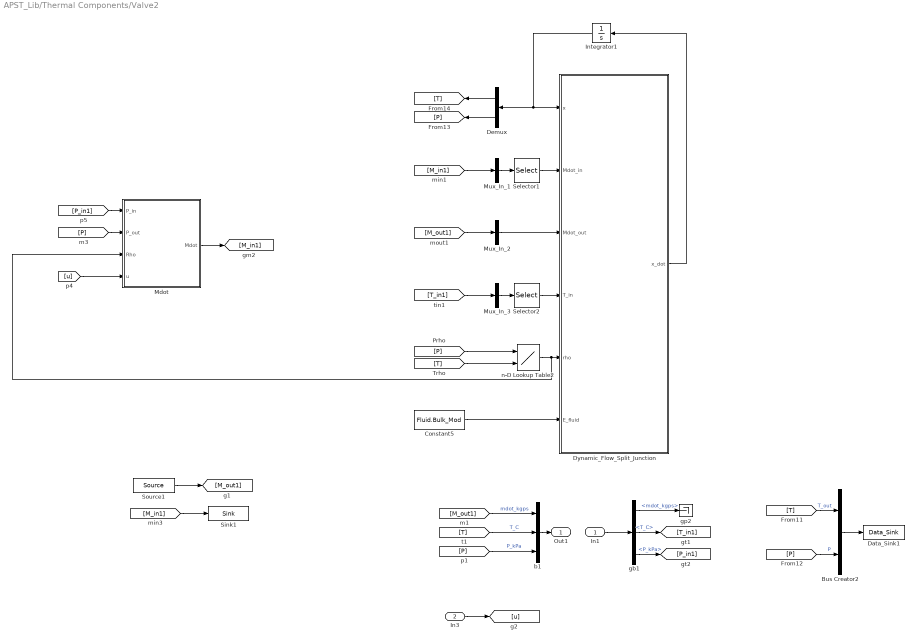
== system APST_Lib/Thermal Components/Valve2 ==
  In1 : Inport
  In3 : Inport  Port=2
  Bus Creator2 : BusCreator  Inputs=2
  Constant5 : Constant  Value=Fluid.Bulk_Mod
  Data_Sink1 : APST_Lib/Support Components/Data_Sink
  Demux : Demux  Outputs=2
  Dynamic_Flow_Split_Junction : MATLAB Function  TreatAsAtomicUnit=on
  Integrator1 : Integrator  InitialCondition=[T_init P_init]
  Mdot : MATLAB Function  TreatAsAtomicUnit=on
  Mux_In_1 : Mux  Inputs=1
  Mux_In_2 : Mux  Inputs=1
  Mux_In_3 : Mux  Inputs=1
  Selector1 : Selector  InputPortWidth=1  IndexOptions=Index vector (dialog)  Indices="[1  ]"  OutputSizes=1
  Selector2 : Selector  InputPortWidth=1  IndexOptions=Index vector (dialog)  Indices="[1  ]"  OutputSizes=1
  Sink1 : APST_Lib/Support Components/Sink
  Source1 : APST_Lib/Support Components/Source
  b1 : BusCreator  Inputs=3
  gb1 : BusSelector  OutputSignals=mdot_kgps,T_C,P_kPa
  gp2 : Terminator
  n-D Lookup Table2 : Lookup_n-D  BreakpointsForDimension1=Fluid.P  BreakpointsForDimension2=Fluid.T  BreakpointsForDimension3=[5, 7]  Table=Fluid.Rho_pt  ExtrapMethod=Clip  UseLastTableValue=on  RndMeth=Simplest  InputSameDT=on
  Out1 : Outport
  wires:
  [u] -> Mdot/4(u)
  In3/1 -> [u]
  Mdot/1(Mdot) -> [M_in1]
  [P] -> Mdot/2(P_out)
  [P_in1] -> Mdot/1(P_in)
  n-D Lookup Table2/1 -> Dynamic_Flow_Split_Junction/5(rho), Mdot/3(Rho)
  Selector2/1 -> Dynamic_Flow_Split_Junction/4(T_in)
  Demux/2 -> [P]
  Demux/1 -> [T]
  [T] -> n-D Lookup Table2/2
  [P] -> n-D Lookup Table2/1
  Constant5/1 -> Dynamic_Flow_Split_Junction/6(E_fluid)
  Selector1/1 -> Dynamic_Flow_Split_Junction/2(Mdot_in)
  Integrator1/1 -> Dynamic_Flow_Split_Junction/1(x), Demux/1
  [P] -> Bus Creator2/2  "P"
  [T] -> Bus Creator2/1  "T_out"
  Bus Creator2/1 -> Data_Sink1/1
  Dynamic_Flow_Split_Junction/1(x_dot) -> Integrator1/1
  [M_in1] -> Sink1/1
  [T_in1] -> Mux_In_3/1
  [M_out1] -> Mux_In_2/1
  [M_in1] -> Mux_In_1/1
  Mux_In_2/1 -> Dynamic_Flow_Split_Junction/3(Mdot_out)
  Mux_In_1/1 -> Selector1/1
  Mux_In_3/1 -> Selector2/1
  gb1/3 -> [P_in1]  "<P_kPa>"
  [P] -> b1/3  "P_kPa"
  In1/1 -> gb1/1
  Source1/1 -> [M_out1]
  gb1/1 -> gp2/1  "<mdot_kgps>"
  [T] -> b1/2  "T_C"
  gb1/2 -> [T_in1]  "<T_C>"
  [M_out1] -> b1/1  "mdot_kgps"
  b1/1 -> Out1/1
